simulink model "boostObserver_old"  (R2020a)
settings: Solver=VariableStepAuto  StartTime=0.0  StopTime=3.2  FixedStep=0.0005  MaxStep=9e-06  RelTol=1e-03  EnableMultiTasking=on
InitFcn:
  | kp=0.01;
  | ki=0.01;
  | 
  | k=2;
  | em=100000000;
  | GE=1/em;
  | GU=k*ki/GE;
  | GCE=k*kp/GU;
model workspace (MAT data in the model file):
  time = 0.8
values from neighbouring files (symbols this model uses):
  A1 = obj.boostConverter.A1    [BoostController.m]    (also in BoostConverter.m = [-obj.R/obj.L 0;0 -1/(obj.Ro*obj.C)]; BuckBoostConverter.m = [-obj.R/obj.L 0;0 -1/(obj.Ro*obj.C)]; obsmc.m = Asigma{1,1}; workspace_atual.mat = [-16.4  0; 0  -3.50877192982])
  A2 = obj.boostConverter.A2    [BoostController.m]    (also in BoostConverter.m = [-obj.R/obj.L -1/obj.L;1/obj.C -1/(obj.Ro*obj.C)]; BuckBoostConverter.m = [-obj.R/obj.L 1/obj.L;-1/obj.C -1/(obj.Ro*obj.C)]; obsmc.m = Asigma{1,2}; workspace_atual.mat = [-16.4  -200; 350.877192982  -3.50877192982])
  AlarmDeadTime = 0.50    (= 0.5)    [BoostFaultSimulation.m]    (also in workspace_atual.mat; workspace_certo.mat)
  B1 = obj.boostConverter.B1    [BoostController.m]    (also in BoostConverter.m = [1/obj.L;0]; BuckBoostConverter.m = [1/obj.L;0]; obsmc.m = Bsigma{1,1}; workspace_atual.mat = [200 0])
  boost_parameters = [obj.Ro,obj.R,obj.L,obj.C,obj.u]'    [BoostConverter.m]    (also in BuckBoostConverter.m; boostResults2Latex.m = boost.parameters(); workspace_atual.mat = [100 0.082 0.005 0.00285 190]; workspace_certo.mat = [100 0.082 0.005 0.00285 190])
  C = 1e-3    (= 0.001)    [boostResults2Latex.m]
  CiL = [0 1]    [workspace_atual.mat]    (also in workspace_certo.mat)
  Cmatrix = [1  0; 0  1]    [workspace_atual.mat]    (also in workspace_certo.mat)
  CVc = [1 0]    [workspace_atual.mat]    (also in workspace_certo.mat)
  D1 = [1  0; 0  1]    [workspace_atual.mat]    (also in workspace_certo.mat)
  FaultClass = 0    [BoostFaultSimulation.m]    (also in workspace_atual.mat = 1; workspace_certo.mat = 1)
  iLFaultSwitch = 0    [BoostFaultSimulation.m]    (also in workspace_atual.mat; workspace_certo.mat)
  iLFaultTime = 1.70    (= 1.7)    [BoostFaultSimulation.m]    (also in workspace_atual.mat; workspace_certo.mat)
  iLGainFaultFactor = 15    [BoostFaultSimulation.m]    (also in workspace_atual.mat; workspace_certo.mat)
  iLNoiseFaultSwitch = 0    [BoostFaultSimulation.m]    (also in workspace_atual.mat; workspace_certo.mat)
  iLNoiseTime = 1.70    (= 1.7)    [BoostFaultSimulation.m]    (also in workspace_atual.mat; workspace_certo.mat)
  Jth = 2000    [workspace_atual.mat]    (also in workspace_certo.mat)
  L = 1e-3    (= 0.001)    [boostResults2Latex.m]    (also in obsmc.m = sdpvar(3,1,'full'))
  LoadAddResistor = obj.LoadAddFactor*obj.Ro    [BoostFaultSimulation.m]    (also in workspace_atual.mat = 30; workspace_certo.mat = 30)
  LoadAddSignalSwitch = 1    [BoostFaultSimulation.m]    (also in workspace_atual.mat; workspace_certo.mat)
  LoadAddSwitch = 0    [BoostFaultSimulation.m]    (also in workspace_atual.mat; workspace_certo.mat)
  LoadAddTime = 0.90    (= 0.9)    [BoostFaultSimulation.m]    (also in workspace_atual.mat; workspace_certo.mat)
  LoadRemoveResistor = obj.Ro*(1-obj.LoadRemoveFactor)/(obj.LoadRemoveFactor)    [BoostFaultSimulation.m]    (also in workspace_atual.mat = 233.333333333; workspace_certo.mat = 233.333333333)
  LoadRemoveSignalSwitch = 1    [BoostFaultSimulation.m]    (also in workspace_atual.mat; workspace_certo.mat)
  LoadRemoveSwitch = 0    [BoostFaultSimulation.m]    (also in workspace_atual.mat; workspace_certo.mat)
  LoadRemoveTime = 0.90    (= 0.9)    [BoostFaultSimulation.m]    (also in workspace_atual.mat; workspace_certo.mat)
  LobsiL = [1737913.15707 66180.0912281]    [workspace_atual.mat]    (also in workspace_certo.mat)
  LobsVc = [61200 1]    [workspace_atual.mat]    (also in workspace_certo.mat)
  ObsEp = 70    [workspace_atual.mat]    (also in workspace_certo.mat)
  R = 0.1    [boostResults2Latex.m]    (also in workspace_atual.mat = 0.082; workspace_certo.mat = 0.082)
  ReconfigDelay = 0    [BoostFaultSimulation.m]    (also in workspace_atual.mat = 0.2; workspace_certo.mat = 0.2)
  ReconfigSwitch = 0    [BoostFaultSimulation.m]    (also in workspace_atual.mat; workspace_certo.mat)
  ReconfigTime = 1.707    [BoostFaultSimulation.m]    (also in workspace_atual.mat; workspace_certo.mat)
  rho = 5    [workspace_atual.mat]    (also in workspace_certo.mat)
  RMSfrequency = 47.61    [BoostFaultSimulation.m]    (also in workspace_atual.mat; workspace_certo.mat)
  Ro = 100    [BoostFaultSimulation.m]    (also in boostResults2Latex.m = 10; workspace_atual.mat; workspace_certo.mat)
  Smep = 80    [workspace_atual.mat]    (also in workspace_certo.mat)
  SourceAddSignalSwitch = 1    [BoostFaultSimulation.m]    (also in workspace_atual.mat; workspace_certo.mat)
  SourceAddSwitch = 0    [BoostFaultSimulation.m]    (also in workspace_atual.mat; workspace_certo.mat)
  SourceAddTime = 0.90    (= 0.9)    [BoostFaultSimulation.m]    (also in workspace_atual.mat; workspace_certo.mat)
  SourceAddVoltage = obj.SourceAddFactor*obj.u    [BoostFaultSimulation.m]    (also in workspace_atual.mat = 19; workspace_certo.mat = 19)
  SourceRemoveSignalSwitch = 1    [BoostFaultSimulation.m]    (also in workspace_atual.mat; workspace_certo.mat)
  SourceRemoveSwitch = 0    [BoostFaultSimulation.m]    (also in workspace_atual.mat; workspace_certo.mat)
  SourceRemoveTime = 0.90    (= 0.9)    [BoostFaultSimulation.m]    (also in workspace_atual.mat; workspace_certo.mat)
  SourceRemoveVoltage = obj.SourceRemoveFactor*obj.u    [BoostFaultSimulation.m]    (also in workspace_atual.mat = 19; workspace_certo.mat = 19)
  ueq = 0.5    [workspace_atual.mat]    (also in workspace_certo.mat)
  VcFaultSwitch = 0    [BoostFaultSimulation.m]    (also in workspace_atual.mat; workspace_certo.mat)
  VcFaultTime = 1.70    (= 1.7)    [BoostFaultSimulation.m]    (also in workspace_atual.mat; workspace_certo.mat)
  VcGainFaultFactor = 15    [BoostFaultSimulation.m]    (also in workspace_atual.mat; workspace_certo.mat)
  VcNoiseFaultSwitch = 0    [BoostFaultSimulation.m]    (also in workspace_atual.mat; workspace_certo.mat)
  VcNoiseTime = 1.70    (= 1.7)    [BoostFaultSimulation.m]    (also in workspace_atual.mat; workspace_certo.mat)
  ve = 380    [BoostFaultSimulation.m]    (also in boostResults2Latex.m = 100; workspace_atual.mat; workspace_certo.mat)
  x_e = [ie;ve]    [BoostConverter.m]    (also in BuckBoostConverter.m)
  xe = obj.boostConverter.equilibriumstate(ve)    [BoostController.m]    (also in workspace_atual.mat = [7.62509288104 380]; workspace_certo.mat = [7.62509288104 380])
undefined symbols (not defined in the file or in its folder): Atilde1, Atilde2, Ctilde1, Dtilde1, Dtilde2, F, G, MAXnet, MINnet
libraries: neural x74, powerlib x70, dspstat3 x16, simulink x9, powerlib_meascontrol x7, dspmtrx3 x7, dspmathops x3
(part 4 of 7)

== system boostObserver_old/reset/D(f_s)/Subsystem ==
  input : Inport
  FaultStep : Inport  Port=2
  NoiseStep : Inport  Port=3
  FaultSwtich : Inport  Port=4
  NoiseFaultSwitch : Inport  Port=5
  FaultFactor : Inport  Port=6
  Constant11 : Constant  Value=0
  Constant9 : Constant  Value=0
  Product : Product
  Subsystem : Subsystem
  Switch{9..11,13} (4 alike) : Switch  Criteria=u2 ~= 0
  iLFault Switch : MultiPortSwitch  DataPortOrder=Zero-based contiguous  DataPortForDefault=Additional data port  zeroidx=on
  output : Outport
  wires:
  input/1 -> Product/1, Switch11/3, Switch10/3, iLFault Switch/2, iLFault Switch/5
  Constant9/1 -> Switch10/1
  Switch13/1 -> Switch9/2
  Switch9/1 -> output/1
  Switch11/1 -> iLFault Switch/4
  Constant11/1 -> Switch13/3
  iLFault Switch/1 -> Switch9/3, Subsystem/1(input)
  Switch10/1 -> iLFault Switch/3
  FaultStep/1 -> Switch10/2, Switch11/2
  NoiseStep/1 -> Switch13/1
  FaultSwtich/1 -> iLFault Switch/1
  NoiseFaultSwitch/1 -> Switch13/2
  Product/1 -> Switch11/1
  FaultFactor/1 -> Product/2
  Subsystem/1(noiseOutput) -> Switch9/1

== system boostObserver_old/reset/D(f_s)/Subsystem2 ==
  input : Inport
  FaultStep : Inport  Port=2
  NoiseStep : Inport  Port=3
  FaultSwtich : Inport  Port=4
  NoiseFaultSwitch : Inport  Port=5
  FaultFactor : Inport  Port=6
  Constant11 : Constant  Value=0
  Constant9 : Constant  Value=0
  Product : Product
  Subsystem : Subsystem
  Switch10 : Switch  Criteria=u2 ~= 0
  Switch11 : Switch  Criteria=u2 ~= 0
  Switch13 : Switch  Criteria=u2 ~= 0
  Switch9 : Switch  Criteria=u2 ~= 0  ZeroCross=off
  iLFault Switch : MultiPortSwitch  DataPortOrder=Zero-based contiguous  DataPortForDefault=Additional data port  zeroidx=on
  output : Outport
  wires:
  input/1 -> Product/1, Switch11/3, iLFault Switch/2, Switch10/3, iLFault Switch/5
  Constant9/1 -> Switch10/1
  Switch13/1 -> Switch9/2
  Switch9/1 -> output/1
  Switch11/1 -> iLFault Switch/4
  Constant11/1 -> Switch13/3
  iLFault Switch/1 -> Switch9/3, Subsystem/1(input)
  Switch10/1 -> iLFault Switch/3
  FaultStep/1 -> Switch11/2, Switch10/2
  NoiseStep/1 -> Switch13/1
  FaultSwtich/1 -> iLFault Switch/1
  NoiseFaultSwitch/1 -> Switch13/2
  FaultFactor/1 -> Product/2
  Product/1 -> Switch11/1
  Subsystem/1(noiseOutput) -> Switch9/1

== system boostObserver_old/reset/ErrorGenerator/If Action Subsystem ==
  e_y : Inport
  Action Port : ActionPort  ActionPortLabel=if(u1 ~= 0)
  Matrix Multiply : Product  Multiplication=Matrix(*)
  Matrix Multiply1 : Product
  Matrizes A1 : Constant  Value=rho
  Matrizes A2 : Constant  Value=F
  Normalization : dspmathops/Normalization  NormType=2-norm  Bias=1e-10  NormOver=Each column  Dimension=1  roundingMode=Floor  overflowMode=off  accumDataTypeStr=Inherit: Same as product output  accumLastDataTypeStr=Inherit: Same as product output  outputDataTypeStr=Inherit: Same as product output  outputMin=[]  outputMax=[]  outputLastDataTypeStr=Inherit: Same as product output
  v : Outport
  wires:
  Matrix Multiply/1 -> Normalization/1
  Matrizes A2/1 -> Matrix Multiply/1
  Normalization/1 -> Matrix Multiply1/2
  e_y/1 -> Matrix Multiply/2
  Matrizes A1/1 -> Matrix Multiply1/1
  Matrix Multiply1/1 -> v/1

== system boostObserver_old/reset/ErrorGenerator/If Action Subsystem1 ==
  e_y : Inport
  Action Port : ActionPort  ActionPortLabel=else
  v : Outport
  wires:
  e_y/1 -> v/1

== system boostObserver_old/reset/Fault Identification Neural Netowrk/Pattern Recognition Neural Network2 ==
  Input : Inport  PortDimensions=3
      mask Display: e = 0.06;c1 = [120 230 180]/255;c2 = ([120 230 180]+0)/(256+128);c3 = ([120 230 180]+128)/(256+128);patch([0 1 1 0],[0 0 1 1],c1);patch([0 1 1 1-e 1-e 0+e],[0 0 1 1-e 0+e 0+e],c2);patch([0 0 1 1-e 0+e 0+e],[0 1 1 1-e 1-e 0+e],c3);plot([0 1 1 0 0],[0 0 1 1 0]);
  Layer 1 : Subsystem
      mask Display: e = 0.06;c1 = [120 150 230]/255;c2 = ([120 150 230]+0)/383;c3 = ([120 150 230]+128)/383;patch([0 1 1 0],[0 0 1 1],c1);patch([0 1 1 1-e 1-e 0+e],[0 0 1 1-e 0+e 0+e],c2);patch([0 0 1 1-e 0+e 0+e],[0 1 1 1-e 1-e 0+e],c3);plot([0 1 1 0 0],[0 0 1 1 0]);
  Layer 2 : Subsystem
      mask Display: e = 0.06;c1 = [120 150 230]/255;c2 = ([120 150 230]+0)/383;c3 = ([120 150 230]+128)/383;patch([0 1 1 0],[0 0 1 1],c1);patch([0 1 1 1-e 1-e 0+e],[0 0 1 1-e 0+e 0+e],c2);patch([0 0 1 1-e 0+e 0+e],[0 1 1 1-e 1-e 0+e],c3);plot([0 1 1 0 0],[0 0 1 1 0]);
  Process Input 1 : Subsystem
      mask Display: e = 0.06;c1 = [120 150 230]/255;c2 = ([120 150 230]+0)/383;c3 = ([120 150 230]+128)/383;patch([0 1 1 0],[0 0 1 1],c1);patch([0 1 1 1-e 1-e 0+e],[0 0 1 1-e 0+e 0+e],c2);patch([0 0 1 1-e 0+e 0+e],[0 1 1 1-e 1-e 0+e],c3);plot([0 1 1 0 0],[0 0 1 1 0]);
  Process Output 1 : Subsystem
      mask Display: e = 0.06;c1 = [120 150 230]/255;c2 = ([120 150 230]+0)/383;c3 = ([120 150 230]+128)/383;patch([0 1 1 0],[0 0 1 1],c1);patch([0 1 1 1-e 1-e 0+e],[0 0 1 1-e 0+e 0+e],c2);patch([0 0 1 1-e 0+e 0+e],[0 1 1 1-e 1-e 0+e],c3);plot([0 1 1 0 0],[0 0 1 1 0]);
  Output : Outport  InitialOutput=[0;0;0;0;0]
      mask Display: e = 0.06;c1 = [120 230 180]/255;c2 = ([120 230 180]+0)/(256+128);c3 = ([120 230 180]+128)/(256+128);patch([0 1 1 0],[0 0 1 1],c1);patch([0 1 1 1-e 1-e 0+e],[0 0 1 1-e 0+e 0+e],c2);patch([0 0 1 1-e 0+e 0+e],[0 1 1 1-e 1-e 0+e],c3);plot([0 1 1 0 0],[0 0 1 1 0]);
  wires:
  Input/1 -> Process Input 1/1(x)
  Process Output 1/1(y) -> Output/1
  Process Input 1/1(p) -> Layer 1/1("p{1}")
  Layer 1/1("a{1}") -> [feedback1]
  [feedback1] -> Layer 2/1("a{1} ")
  Layer 2/1("a{2}") -> Process Output 1/1(a)

== system boostObserver_old/reset/Fault Identification Neural Netowrk/Pattern Recognition Neural Network3 ==
  Input : Inport  PortDimensions=3
      mask Display: e = 0.06;c1 = [120 230 180]/255;c2 = ([120 230 180]+0)/(256+128);c3 = ([120 230 180]+128)/(256+128);patch([0 1 1 0],[0 0 1 1],c1);patch([0 1 1 1-e 1-e 0+e],[0 0 1 1-e 0+e 0+e],c2);patch([0 0 1 1-e 0+e 0+e],[0 1 1 1-e 1-e 0+e],c3);plot([0 1 1 0 0],[0 0 1 1 0]);
  Layer 1 : Subsystem
      mask Display: e = 0.06;c1 = [120 150 230]/255;c2 = ([120 150 230]+0)/383;c3 = ([120 150 230]+128)/383;patch([0 1 1 0],[0 0 1 1],c1);patch([0 1 1 1-e 1-e 0+e],[0 0 1 1-e 0+e 0+e],c2);patch([0 0 1 1-e 0+e 0+e],[0 1 1 1-e 1-e 0+e],c3);plot([0 1 1 0 0],[0 0 1 1 0]);
  Layer 2 : Subsystem
      mask Display: e = 0.06;c1 = [120 150 230]/255;c2 = ([120 150 230]+0)/383;c3 = ([120 150 230]+128)/383;patch([0 1 1 0],[0 0 1 1],c1);patch([0 1 1 1-e 1-e 0+e],[0 0 1 1-e 0+e 0+e],c2);patch([0 0 1 1-e 0+e 0+e],[0 1 1 1-e 1-e 0+e],c3);plot([0 1 1 0 0],[0 0 1 1 0]);
  Process Input 1 : Subsystem
      mask Display: e = 0.06;c1 = [120 150 230]/255;c2 = ([120 150 230]+0)/383;c3 = ([120 150 230]+128)/383;patch([0 1 1 0],[0 0 1 1],c1);patch([0 1 1 1-e 1-e 0+e],[0 0 1 1-e 0+e 0+e],c2);patch([0 0 1 1-e 0+e 0+e],[0 1 1 1-e 1-e 0+e],c3);plot([0 1 1 0 0],[0 0 1 1 0]);
  Process Output 1 : Subsystem
      mask Display: e = 0.06;c1 = [120 150 230]/255;c2 = ([120 150 230]+0)/383;c3 = ([120 150 230]+128)/383;patch([0 1 1 0],[0 0 1 1],c1);patch([0 1 1 1-e 1-e 0+e],[0 0 1 1-e 0+e 0+e],c2);patch([0 0 1 1-e 0+e 0+e],[0 1 1 1-e 1-e 0+e],c3);plot([0 1 1 0 0],[0 0 1 1 0]);
  Output : Outport  InitialOutput=[0;0;0;0;0]
      mask Display: e = 0.06;c1 = [120 230 180]/255;c2 = ([120 230 180]+0)/(256+128);c3 = ([120 230 180]+128)/(256+128);patch([0 1 1 0],[0 0 1 1],c1);patch([0 1 1 1-e 1-e 0+e],[0 0 1 1-e 0+e 0+e],c2);patch([0 0 1 1-e 0+e 0+e],[0 1 1 1-e 1-e 0+e],c3);plot([0 1 1 0 0],[0 0 1 1 0]);
  wires:
  Input/1 -> Process Input 1/1(x)
  Process Output 1/1(y) -> Output/1
  Process Input 1/1(p) -> Layer 1/1("p{1}")
  Layer 1/1("a{1}") -> [feedback1]
  [feedback1] -> Layer 2/1("a{1} ")
  Layer 2/1("a{2}") -> Process Output 1/1(a)

== system boostObserver_old/reset/If Action Subsystem1/GetInitialTime ==
  Clock : Inport
  Constant2 : Constant  Value=0
  Constant3 : Constant
  Constant4 : Constant  Value=0
  Edge Detector : powerlib_meascontrol/Logic/Edge Detector  model=Rising  ic=0  Ts=0
      settings: SourceProductBaseCode=PS
  If : If
  If Action Subsystem : Subsystem  TreatAsAtomicUnit=on
  If Action Subsystem1 : Subsystem  TreatAsAtomicUnit=on
  Memory : Memory
  Merge : Merge
  Switch : Switch  Criteria=u2 > Threshold
  Switch1 : Switch  Criteria=u2 > Threshold
  InitialTime : Outport
  wires:
  If/2 -> If Action Subsystem1/Action
  Memory/1 -> Switch1/3
  Constant3/1 -> Switch/1
  Switch1/1 -> InitialTime/1, Memory/1
  Merge/1 -> Switch1/2, Switch1/1
  Constant4/1 -> Switch/3
  Switch/1 -> If/1
  Constant2/1 -> If Action Subsystem1/1(In1)
  Clock/1 -> [Clock], Edge Detector/1
  If Action Subsystem/1(Out1) -> Merge/2
  Edge Detector/1 -> Switch/2
  [Clock] -> If Action Subsystem/1(In1)
  If/1 -> If Action Subsystem/Action
  If Action Subsystem1/1(Out1) -> Merge/1

== system boostObserver_old/reset/If Action Subsystem4/GetInitialTime ==
  Clock : Inport
  Constant2 : Constant  Value=0
  Constant3 : Constant
  Constant4 : Constant  Value=0
  Edge Detector : powerlib_meascontrol/Logic/Edge Detector  model=Rising  ic=0  Ts=0
      settings: SourceProductBaseCode=PS
  If : If
  If Action Subsystem : Subsystem  TreatAsAtomicUnit=on
  If Action Subsystem1 : Subsystem  TreatAsAtomicUnit=on
  Memory : Memory
  Merge : Merge
  Switch : Switch  Criteria=u2 > Threshold
  Switch1 : Switch  Criteria=u2 > Threshold
  InitialTime : Outport
  wires:
  If/2 -> If Action Subsystem1/Action
  Memory/1 -> Switch1/3
  Constant3/1 -> Switch/1
  Switch1/1 -> InitialTime/1, Memory/1
  Merge/1 -> Switch1/2, Switch1/1
  Constant4/1 -> Switch/3
  Switch/1 -> If/1
  Constant2/1 -> If Action Subsystem1/1(In1)
  Clock/1 -> [Clock], Edge Detector/1
  If Action Subsystem/1(Out1) -> Merge/2
  Edge Detector/1 -> Switch/2
  [Clock] -> If Action Subsystem/1(In1)
  If/1 -> If Action Subsystem/Action
  If Action Subsystem1/1(Out1) -> Merge/1

== system boostObserver_old/reset/Sliding Mode Observer 5/ObserverDynamics ==
  ey : Inport
  v : Inport  Port=2
  sigma : Inport  Port=3
  Gain : Gain  Gain=Atilde1  Multiplication=Matrix(K*u)
  Gain1 : Gain  Gain=G  Multiplication=Matrix(K*u)
  Gain3 : Gain  Gain=Dtilde1  Multiplication=Matrix(K*u)
  Gain5 : Gain  Gain=Atilde2  Multiplication=Matrix(K*u)
  Gain7 : Gain  Gain=Dtilde2  Multiplication=Matrix(K*u)
  Integral : Subsystem
  Sum : Sum  Inputs=|+++
  Sum1 : Sum  Inputs=|+++
  Switch1 : Switch  Criteria=u2 > Threshold
  e_tilde_hat : Outport
  wires:
  sigma/1 -> Switch1/2
  Switch1/1 -> Integral/1(e_hat_dot)  "v"
  Integral/1(e_hat) -> Gain/1, e_tilde_hat/1, Gain5/1
  ey/1 -> Gain1/1
  v/1 -> Gain7/1, Gain3/1
  Sum1/1 -> Switch1/3
  Sum/1 -> Switch1/1
  Gain7/1 -> Sum1/2
  Gain5/1 -> Sum1/3
  Gain3/1 -> Sum/1
  Gain1/1 -> Sum1/1, Sum/2
  Gain/1 -> Sum/3

== system boostObserver_old/reset/Subsystem/SlidingSurface ==
  S : Inport
  ep : Inport  Port=2
  Abs : Abs  ZeroCross=off
  GreaterThan : RelationalOperator  Operator=>  OutDataTypeStr=boolean  RndMeth=Simplest
  If : If  IfExpression=u1 ~= 0
  If Action Subsystem : Subsystem  TreatAsAtomicUnit=on
  If Action Subsystem2 : Subsystem  TreatAsAtomicUnit=on
  Merge1 : Merge
  d : Outport
  wires:
  If Action Subsystem2/1(d) -> Merge1/2
  [S] -> If Action Subsystem/1(S), If Action Subsystem2/1(S)
  If/2 -> If Action Subsystem2/Action
  If/1 -> If Action Subsystem/Action
  [ep] -> If Action Subsystem2/2(ep)
  S/1 -> [S], Abs/1
  If Action Subsystem/1(d) -> Merge1/1
  Abs/1 -> GreaterThan/1
  GreaterThan/1 -> If/1
  Merge1/1 -> d/1
  ep/1 -> [ep], GreaterThan/2

== system boostObserver_old/reset/Subsystem1/SlidingSurface ==
  S : Inport
  ep : Inport  Port=2
  Abs : Abs  ZeroCross=off
  GreaterThan : RelationalOperator  Operator=>  OutDataTypeStr=boolean  RndMeth=Simplest
  If : If  IfExpression=u1 ~= 0
  If Action Subsystem : Subsystem  TreatAsAtomicUnit=on
  If Action Subsystem2 : Subsystem  TreatAsAtomicUnit=on
  Merge1 : Merge
  d : Outport
  wires:
  If Action Subsystem2/1(d) -> Merge1/2
  [S] -> If Action Subsystem/1(S), If Action Subsystem2/1(S)
  If/2 -> If Action Subsystem2/Action
  If/1 -> If Action Subsystem/Action
  [ep] -> If Action Subsystem2/2(ep)
  S/1 -> [S], Abs/1
  If Action Subsystem/1(d) -> Merge1/1
  Abs/1 -> GreaterThan/1
  GreaterThan/1 -> If/1
  Merge1/1 -> d/1
  ep/1 -> [ep], GreaterThan/2

== system boostObserver_old/reset/Subsystem9/Residual Generator1 ==
  e_y : Inport
  Moving RMS : dspstat3/Moving RMS  Method=Sliding window  ForgettingFactorPort=off  SpecifyWindowLength=on  WindowLength=RMSfrequency  ForgettingFactor=0.9  SimulateUsing=Code generation
      settings: SourceProductBaseCode=DS
  RMS : Outport
  wires:
  e_y/1 -> Moving RMS/1
  Moving RMS/1 -> RMS/1

== system boostObserver_old/reset/Subsystem9/Residual Generator2 ==
  e_y : Inport
  Moving RMS : dspstat3/Moving RMS  Method=Sliding window  ForgettingFactorPort=off  SpecifyWindowLength=on  WindowLength=RMSfrequency  ForgettingFactor=0.9  SimulateUsing=Code generation
      settings: SourceProductBaseCode=DS
  RMS : Outport
  wires:
  e_y/1 -> Moving RMS/1
  Moving RMS/1 -> RMS/1

== system boostObserver_old/reset/Vc OBserver/calc_x_hat ==
  sigma : Inport
  rsign : Inport  Port=2
  Lobs : Inport  Port=3
  Gain : Gain  Gain=A1  Multiplication=Matrix(K*u)
  Gain5 : Gain  Gain=A2  Multiplication=Matrix(K*u)
  Integral : Subsystem
  Matrix Multiply : Product  Multiplication=Matrix(*)
  MatrizesA8 : Constant  Value=B1*u
  Scope1 : Scope
  Sum : Sum  Inputs=|+++
  Sum1 : Sum  Inputs=|+++
  Switch1 : Switch  Criteria=u2 ~= 0
  x_hat : Outport
  wires:
  sigma/1 -> Switch1/2
  Switch1/1 -> Integral/1(x_hat_dot)  "v"
  Integral/1(x_hat) -> Scope1/1, x_hat/1, Gain/1, Gain5/1
  Sum1/1 -> Switch1/3
  Sum/1 -> Switch1/1
  Gain/1 -> Sum/3
  Gain5/1 -> Sum1/3
  Matrix Multiply/1 -> Sum/2, Sum1/2
  MatrizesA8/1 -> Sum1/1, Sum/1
  Lobs/1 -> Matrix Multiply/1
  rsign/1 -> Matrix Multiply/2

== system boostObserver_old/reset/iL Observer/calc_x_hat ==
  sigma : Inport
  rsign : Inport  Port=2
  Lobs : Inport  Port=3
  Gain : Gain  Gain=A1  Multiplication=Matrix(K*u)
  Gain5 : Gain  Gain=A2  Multiplication=Matrix(K*u)
  Integral : Subsystem
  Matrix Multiply : Product  Multiplication=Matrix(*)
  MatrizesA8 : Constant  Value=B1*u
  Scope1 : Scope
  Sum : Sum  Inputs=|+++
  Sum1 : Sum  Inputs=|+++
  Switch1 : Switch  Criteria=u2 ~= 0
  x_hat : Outport
  wires:
  sigma/1 -> Switch1/2
  Switch1/1 -> Integral/1(x_hat_dot)  "v"
  Integral/1(x_hat) -> Scope1/1, x_hat/1, Gain/1, Gain5/1
  Sum1/1 -> Switch1/3
  Sum/1 -> Switch1/1
  Gain/1 -> Sum/3
  Gain5/1 -> Sum1/3
  Matrix Multiply/1 -> Sum/2, Sum1/2
  MatrizesA8/1 -> Sum1/1, Sum/1
  Lobs/1 -> Matrix Multiply/1
  rsign/1 -> Matrix Multiply/2

== system boostObserver_old/Subsystem/Boost Converter/TipoEntrada/disturbio ==
  Step1 : Step  SampleTime=0
  Step2 : Step  Time=1.1  After=-1  SampleTime=0
  Sum : Sum  Inputs=|++
  disturbio : Outport
  wires:
  Sum/1 -> disturbio/1
  Step2/1 -> Sum/2
  Step1/1 -> Sum/1

== system boostObserver_old/Subsystem/Boost Converter/TipoEntrada/disturbio1 ==
  Step1 : Step  Time=1.2  SampleTime=0
  Step2 : Step  Time=1.4  After=-1  SampleTime=0
  Sum : Sum  Inputs=|++
  disturbio : Outport
  wires:
  Sum/1 -> disturbio/1
  Step2/1 -> Sum/2
  Step1/1 -> Sum/1

== system boostObserver_old/Subsystem/Boost Converter/TipoEntrada/disturbio2 ==
  Step1 : Step  Time=1.2  SampleTime=0
  Step2 : Step  Time=1.4  After=-1  SampleTime=0
  Sum : Sum  Inputs=|++
  disturbio : Outport
  wires:
  Sum/1 -> disturbio/1
  Step2/1 -> Sum/2
  Step1/1 -> Sum/1

== system boostObserver_old/Subsystem/Boost Converter/TipoEntrada/disturbio3 ==
  Step1 : Step  SampleTime=0
  Step2 : Step  Time=1.1  After=-1  SampleTime=0
  Sum : Sum  Inputs=|++
  disturbio : Outport
  wires:
  Sum/1 -> disturbio/1
  Step2/1 -> Sum/2
  Step1/1 -> Sum/1

== system boostObserver_old/Subsystem/Controlador1/SlidingSurface/If Action Subsystem ==
  S : Inport
  Action Port : ActionPort  ActionPortLabel=if(u1 ~= 0)
  Sign : Signum
  d : Outport
  wires:
  S/1 -> Sign/1
  Sign/1 -> d/1

== system boostObserver_old/Subsystem/Controlador1/SlidingSurface/If Action Subsystem2 ==
  S : Inport
  ep : Inport  Port=2
  Action Port : ActionPort  ActionPortLabel=else
  Divide : Product  Inputs=*/
  d : Outport
  wires:
  S/1 -> Divide/1
  ep/1 -> Divide/2
  Divide/1 -> d/1

== system boostObserver_old/Subsystem/D(f_s)/Subsystem/Subsystem ==
  input : Inport
  Add : Sum
  Band-Limited White Noise : simulink/Sources/Band-Limited White Noise  Cov=[0.1]  Ts=0.1  seed=[23341]
  noiseOutput : Outport
  wires:
  Band-Limited White Noise/1 -> Add/1
  Add/1 -> noiseOutput/1
  input/1 -> Add/2

== system boostObserver_old/Subsystem/D(f_s)/Subsystem2/Subsystem ==
  input : Inport
  Add : Sum
  Band-Limited White Noise : simulink/Sources/Band-Limited White Noise  Cov=[0.1]  Ts=0.1  seed=[23341]
  noiseOutput : Outport
  wires:
  Band-Limited White Noise/1 -> Add/1
  Add/1 -> noiseOutput/1
  input/1 -> Add/2

== system boostObserver_old/Subsystem/Fault Identification Neural Netowrk/Pattern Recognition Neural Network1/Layer 1 ==
  "p{1}" : Inport  PortDimensions=3
      mask Display: e = 0.06;c1 = [120 230 180]/255;c2 = ([120 230 180]+0)/(256+128);c3 = ([120 230 180]+128)/(256+128);patch([0 1 1 0],[0 0 1 1],c1);patch([0 1 1 1-e 1-e 0+e],[0 0 1 1-e 0+e 0+e],c2);patch([0 0 1 1-e 0+e 0+e],[0 1 1 1-e 1-e 0+e],c3);plot([0 1 1 0 0],[0 0 1 1 0]);
  Delays 1 : Subsystem
      mask Display: e = 0.06;c1 = [120 150 230]/255;c2 = ([120 150 230]+0)/383;c3 = ([120 150 230]+128)/383;patch([0 1 1 0],[0 0 1 1],c1);patch([0 1 1 1-e 1-e 0+e],[0 0 1 1-e 0+e 0+e],c2);patch([0 0 1 1-e 0+e 0+e],[0 1 1 1-e 1-e 0+e],c3);plot([0 1 1 0 0],[0 0 1 1 0]);disp('0');
  "IW{1,1}" : Subsystem
      mask Display: e = 0.06;c1 = [120 150 230]/255;c2 = ([120 150 230]+0)/383;c3 = ([120 150 230]+128)/383;patch([0 1 1 0],[0 0 1 1],c1);patch([0 1 1 1-e 1-e 0+e],[0 0 1 1-e 0+e 0+e],c2);patch([0 0 1 1-e 0+e 0+e],[0 1 1 1-e 1-e 0+e],c3);plot([0 1 1 0 0],[0 0 1 1 0]);disp('W');
  "b{1}" : Constant  Value=[-3.0907169643136906955760423443280160427093505859375;-8.5532408660313894444016113993711769580841064453125;26.179031484954197850356649723835289478302001953125;0.130591451617109999272514642143505625426769256591796875]
      mask Display: e = 0.06;c1 = [120 150 230]/255;c2 = ([120 150 230]+0)/383;c3 = ([120 150 230]+128)/383;patch([0 1 1 0],[0 0 1 1],c1);patch([0 1 1 1-e 1-e 0+e],[0 0 1 1-e 0+e 0+e],c2);patch([0 0 1 1-e 0+e 0+e],[0 1 1 1-e 1-e 0+e],c3);plot([0 1 1 0 0],[0 0 1 1 0]);disp('b');
  netsum : Sum  Inputs=2  InputSameDT=on  SaturateOnIntegerOverflow=on  OutDataTypeStr=Inherit: Same as first input
      mask Display: e = 0.06;c1 = [120 150 230]/255;c2 = ([120 150 230]+0)/383;c3 = ([120 150 230]+128)/383;patch([0 1 1 0],[0 0 1 1],c1);patch([0 1 1 1-e 1-e 0+e],[0 0 1 1-e 0+e 0+e],c2);patch([0 0 1 1-e 0+e 0+e],[0 1 1 1-e 1-e 0+e],c3);plot([0 1 1 0 0],[0 0 1 1 0]);disp('+');
  tansig : neural/Transfer Functions/tansig
  "a{1}" : Outport  InitialOutput=[0;0;0;0]
      mask Display: e = 0.06;c1 = [120 230 180]/255;c2 = ([120 230 180]+0)/(256+128);c3 = ([120 230 180]+128)/(256+128);patch([0 1 1 0],[0 0 1 1],c1);patch([0 1 1 1-e 1-e 0+e],[0 0 1 1-e 0+e 0+e],c2);patch([0 0 1 1-e 0+e 0+e],[0 1 1 1-e 1-e 0+e],c3);plot([0 1 1 0 0],[0 0 1 1 0]);
  wires:
  "p{1}"/1 -> Delays 1/1("p{1}")
  Delays 1/1("pd{1,1}") -> "IW{1,1}"/1("pd{1,1}")
  "IW{1,1}"/1("iz{1,1}") -> netsum/1
  "b{1}"/1 -> netsum/2
  netsum/1 -> tansig/1
  tansig/1 -> "a{1}"/1

== system boostObserver_old/Subsystem/Fault Identification Neural Netowrk/Pattern Recognition Neural Network1/Layer 2 ==
  "a{1} " : Inport  PortDimensions=4
      mask Display: e = 0.06;c1 = [120 230 180]/255;c2 = ([120 230 180]+0)/(256+128);c3 = ([120 230 180]+128)/(256+128);patch([0 1 1 0],[0 0 1 1],c1);patch([0 1 1 1-e 1-e 0+e],[0 0 1 1-e 0+e 0+e],c2);patch([0 0 1 1-e 0+e 0+e],[0 1 1 1-e 1-e 0+e],c3);plot([0 1 1 0 0],[0 0 1 1 0]);
  Delays 1 : Subsystem
      mask Display: e = 0.06;c1 = [120 150 230]/255;c2 = ([120 150 230]+0)/383;c3 = ([120 150 230]+128)/383;patch([0 1 1 0],[0 0 1 1],c1);patch([0 1 1 1-e 1-e 0+e],[0 0 1 1-e 0+e 0+e],c2);patch([0 0 1 1-e 0+e 0+e],[0 1 1 1-e 1-e 0+e],c3);plot([0 1 1 0 0],[0 0 1 1 0]);disp('0');
  "LW{2,1}" : Subsystem
      mask Display: e = 0.06;c1 = [120 150 230]/255;c2 = ([120 150 230]+0)/383;c3 = ([120 150 230]+128)/383;patch([0 1 1 0],[0 0 1 1],c1);patch([0 1 1 1-e 1-e 0+e],[0 0 1 1-e 0+e 0+e],c2);patch([0 0 1 1-e 0+e 0+e],[0 1 1 1-e 1-e 0+e],c3);plot([0 1 1 0 0],[0 0 1 1 0]);disp('W');
  "b{2}" : Constant  Value=[-2.302427575546979188203522426192648708820343017578125;-5.91134493996858534359262193902395665645599365234375;6.8980698616354221286428582970984280109405517578125;0.77959090259712271464564992129453457891941070556640625;-0.782333279931369585113998255110345780849456787109375]
      mask Display: e = 0.06;c1 = [120 150 230]/255;c2 = ([120 150 230]+0)/383;c3 = ([120 150 230]+128)/383;patch([0 1 1 0],[0 0 1 1],c1);patch([0 1 1 1-e 1-e 0+e],[0 0 1 1-e 0+e 0+e],c2);patch([0 0 1 1-e 0+e 0+e],[0 1 1 1-e 1-e 0+e],c3);plot([0 1 1 0 0],[0 0 1 1 0]);disp('b');
  netsum : Sum  Inputs=2  InputSameDT=on  SaturateOnIntegerOverflow=on  OutDataTypeStr=Inherit: Same as first input
      mask Display: e = 0.06;c1 = [120 150 230]/255;c2 = ([120 150 230]+0)/383;c3 = ([120 150 230]+128)/383;patch([0 1 1 0],[0 0 1 1],c1);patch([0 1 1 1-e 1-e 0+e],[0 0 1 1-e 0+e 0+e],c2);patch([0 0 1 1-e 0+e 0+e],[0 1 1 1-e 1-e 0+e],c3);plot([0 1 1 0 0],[0 0 1 1 0]);disp('+');
  softmax : neural/Transfer Functions/softmax
      settings: SourceProductBaseCode=NN
  "a{2}" : Outport  InitialOutput=[0;0;0;0;0]
      mask Display: e = 0.06;c1 = [120 230 180]/255;c2 = ([120 230 180]+0)/(256+128);c3 = ([120 230 180]+128)/(256+128);patch([0 1 1 0],[0 0 1 1],c1);patch([0 1 1 1-e 1-e 0+e],[0 0 1 1-e 0+e 0+e],c2);patch([0 0 1 1-e 0+e 0+e],[0 1 1 1-e 1-e 0+e],c3);plot([0 1 1 0 0],[0 0 1 1 0]);
  wires:
  "a{1} "/1 -> Delays 1/1("p{2}")
  Delays 1/1("pd{2,1}") -> "LW{2,1}"/1("ad{2,1}")
  "LW{2,1}"/1("lz{2,1}") -> netsum/1
  "b{2}"/1 -> netsum/2
  netsum/1 -> softmax/1
  softmax/1 -> "a{2}"/1

== system boostObserver_old/Subsystem/Fault Identification Neural Netowrk/Pattern Recognition Neural Network1/Process Input 1 ==
  x : Inport  PortDimensions=3
      mask Display: e = 0.06;c1 = [120 230 180]/255;c2 = ([120 230 180]+0)/(256+128);c3 = ([120 230 180]+128)/(256+128);patch([0 1 1 0],[0 0 1 1],c1);patch([0 1 1 1-e 1-e 0+e],[0 0 1 1-e 0+e 0+e],c2);patch([0 0 1 1-e 0+e 0+e],[0 1 1 1-e 1-e 0+e],c3);plot([0 1 1 0 0],[0 0 1 1 0]);
  mapminmax : neural/Processing Functions/mapminmax  xmin=[0;0;-2641.94920061935135890962556005]  xmax=[786.388396902503131968842353672;8926.40391005816127290017902851;8647.99703455211783875711262226]  ymin=-1  ymax=1
  p : Outport  PortDimensions=3
      mask Display: e = 0.06;c1 = [120 230 180]/255;c2 = ([120 230 180]+0)/(256+128);c3 = ([120 230 180]+128)/(256+128);patch([0 1 1 0],[0 0 1 1],c1);patch([0 1 1 1-e 1-e 0+e],[0 0 1 1-e 0+e 0+e],c2);patch([0 0 1 1-e 0+e 0+e],[0 1 1 1-e 1-e 0+e],c3);plot([0 1 1 0 0],[0 0 1 1 0]);
  wires:
  x/1 -> mapminmax/1
  mapminmax/1 -> p/1

== system boostObserver_old/Subsystem/Fault Identification Neural Netowrk/Pattern Recognition Neural Network1/Process Output 1 ==
  a : Inport  PortDimensions=5
      mask Display: e = 0.06;c1 = [120 230 180]/255;c2 = ([120 230 180]+0)/(256+128);c3 = ([120 230 180]+128)/(256+128);patch([0 1 1 0],[0 0 1 1],c1);patch([0 1 1 1-e 1-e 0+e],[0 0 1 1-e 0+e 0+e],c2);patch([0 0 1 1-e 0+e 0+e],[0 1 1 1-e 1-e 0+e],c3);plot([0 1 1 0 0],[0 0 1 1 0]);
  y : Outport  PortDimensions=5
      mask Display: e = 0.06;c1 = [120 230 180]/255;c2 = ([120 230 180]+0)/(256+128);c3 = ([120 230 180]+128)/(256+128);patch([0 1 1 0],[0 0 1 1],c1);patch([0 1 1 1-e 1-e 0+e],[0 0 1 1-e 0+e 0+e],c2);patch([0 0 1 1-e 0+e 0+e],[0 1 1 1-e 1-e 0+e],c3);plot([0 1 1 0 0],[0 0 1 1 0]);
  wires:
  a/1 -> y/1

== system boostObserver_old/Subsystem/Sliding Mode Observer 5/ObserverDynamics/Integral ==
  e_hat_dot : Inport
  Ground{1..4} (4 alike) : Ground
  IC : InitialCondition  Value=[-xe;0;0]
  Integrator5 : Integrator  InitialConditionSource=external  InitialCondition=[-x_e; 0; 0]
  Mux : Mux
  e_hat : Outport
  wires:
  e_hat_dot/1 -> Integrator5/1
  Integrator5/1 -> e_hat/1
  IC/1 -> Integrator5/2
  Ground1/1 -> Mux/1
  Ground2/1 -> Mux/2
  Ground3/1 -> Mux/3
  Ground4/1 -> Mux/4
  Mux/1 -> IC/1

== system boostObserver_old/Subsystem/Subsystem/SlidingSurface/If Action Subsystem ==
  S : Inport
  Action Port : ActionPort  ActionPortLabel=if(u1 ~= 0)
  Sign : Signum
  d : Outport
  wires:
  S/1 -> Sign/1
  Sign/1 -> d/1

== system boostObserver_old/Subsystem/Subsystem/SlidingSurface/If Action Subsystem2 ==
  S : Inport
  ep : Inport  Port=2
  Action Port : ActionPort  ActionPortLabel=else
  Divide : Product  Inputs=*/
  d : Outport
  wires:
  S/1 -> Divide/1
  ep/1 -> Divide/2
  Divide/1 -> d/1

== system boostObserver_old/Subsystem/Subsystem1/SlidingSurface/If Action Subsystem ==
  S : Inport
  Action Port : ActionPort  ActionPortLabel=if(u1 ~= 0)
  Sign : Signum
  d : Outport
  wires:
  S/1 -> Sign/1
  Sign/1 -> d/1

== system boostObserver_old/Subsystem/Subsystem1/SlidingSurface/If Action Subsystem2 ==
  S : Inport
  ep : Inport  Port=2
  Action Port : ActionPort  ActionPortLabel=else
  Divide : Product  Inputs=*/
  d : Outport
  wires:
  S/1 -> Divide/1
  ep/1 -> Divide/2
  Divide/1 -> d/1

== system boostObserver_old/Subsystem/Vc OBserver/calc_x_hat/Integral ==
  x_hat_dot : Inport
  Ground1 : Ground
  Ground2 : Ground
  IC : InitialCondition  Value=[0;0]
  Integrator1 : Integrator  InitialConditionSource=external  InitialCondition=[-x_e; 0; 0]
  Mux : Mux  Inputs=2
  x_hat : Outport
  wires:
  x_hat_dot/1 -> Integrator1/1
  Integrator1/1 -> x_hat/1
  IC/1 -> Integrator1/2
  Ground1/1 -> Mux/1
  Ground2/1 -> Mux/2
  Mux/1 -> IC/1

== system boostObserver_old/Subsystem/iL Observer/calc_x_hat/Integral ==
  x_hat_dot : Inport
  Ground : Ground
  Ground1 : Ground
  IC : InitialCondition  Value=[0;0]
  Integrator1 : Integrator  InitialConditionSource=external  InitialCondition=[-x_e; 0; 0]
  Mux : Mux  Inputs=2
  x_hat : Outport
  wires:
  x_hat_dot/1 -> Integrator1/1
  Integrator1/1 -> x_hat/1
  Mux/1 -> IC/1
  Ground/1 -> Mux/1
  Ground1/1 -> Mux/2
  IC/1 -> Integrator1/2

== system boostObserver_old/Subsystem3/Boost Converter/TipoEntrada/disturbio ==
  Step1 : Step  SampleTime=0
  Step2 : Step  Time=1.1  After=-1  SampleTime=0
  Sum : Sum  Inputs=|++
  disturbio : Outport
  wires:
  Sum/1 -> disturbio/1
  Step2/1 -> Sum/2
  Step1/1 -> Sum/1

== system boostObserver_old/Subsystem3/Boost Converter/TipoEntrada/disturbio1 ==
  Step1 : Step  Time=1.2  SampleTime=0
  Step2 : Step  Time=1.4  After=-1  SampleTime=0
  Sum : Sum  Inputs=|++
  disturbio : Outport
  wires:
  Sum/1 -> disturbio/1
  Step2/1 -> Sum/2
  Step1/1 -> Sum/1

== system boostObserver_old/Subsystem3/Boost Converter/TipoEntrada/disturbio2 ==
  Step1 : Step  Time=1.2  SampleTime=0
  Step2 : Step  Time=1.4  After=-1  SampleTime=0
  Sum : Sum  Inputs=|++
  disturbio : Outport
  wires:
  Sum/1 -> disturbio/1
  Step2/1 -> Sum/2
  Step1/1 -> Sum/1

== system boostObserver_old/Subsystem3/Boost Converter/TipoEntrada/disturbio3 ==
  Step1 : Step  SampleTime=0
  Step2 : Step  Time=1.1  After=-1  SampleTime=0
  Sum : Sum  Inputs=|++
  disturbio : Outport
  wires:
  Sum/1 -> disturbio/1
  Step2/1 -> Sum/2
  Step1/1 -> Sum/1

== system boostObserver_old/Subsystem3/Controlador1/SlidingSurface/If Action Subsystem ==
  S : Inport
  Action Port : ActionPort
  Sign : Signum
  d : Outport
  wires:
  S/1 -> Sign/1
  Sign/1 -> d/1

== system boostObserver_old/Subsystem3/Controlador1/SlidingSurface/If Action Subsystem2 ==
  S : Inport
  ep : Inport  Port=2
  Action Port : ActionPort
  Divide : Product  Inputs=*/
  d : Outport
  wires:
  S/1 -> Divide/1
  ep/1 -> Divide/2
  Divide/1 -> d/1

== system boostObserver_old/Subsystem3/D(f_s)/Subsystem/Subsystem ==
  input : Inport
  Add : Sum
  Band-Limited White Noise : simulink/Sources/Band-Limited White Noise  Cov=[0.1]  Ts=0.1  seed=[23341]
  noiseOutput : Outport
  wires:
  Band-Limited White Noise/1 -> Add/1
  Add/1 -> noiseOutput/1
  input/1 -> Add/2

== system boostObserver_old/Subsystem3/D(f_s)/Subsystem2/Subsystem ==
  input : Inport
  Add : Sum
  Band-Limited White Noise : simulink/Sources/Band-Limited White Noise  Cov=[0.1]  Ts=0.1  seed=[23341]
  noiseOutput : Outport
  wires:
  Band-Limited White Noise/1 -> Add/1
  Add/1 -> noiseOutput/1
  input/1 -> Add/2

== system boostObserver_old/Subsystem3/Fault Identification Neural Netowrk/Pattern Recognition Neural Network/Layer 1 ==
  "p{1}" : Inport  PortDimensions=3
      mask Display: e = 0.06;c1 = [120 230 180]/255;c2 = ([120 230 180]+0)/(256+128);c3 = ([120 230 180]+128)/(256+128);patch([0 1 1 0],[0 0 1 1],c1);patch([0 1 1 1-e 1-e 0+e],[0 0 1 1-e 0+e 0+e],c2);patch([0 0 1 1-e 0+e 0+e],[0 1 1 1-e 1-e 0+e],c3);plot([0 1 1 0 0],[0 0 1 1 0]);
  Delays 1 : Subsystem
      mask Display: e = 0.06;c1 = [120 150 230]/255;c2 = ([120 150 230]+0)/383;c3 = ([120 150 230]+128)/383;patch([0 1 1 0],[0 0 1 1],c1);patch([0 1 1 1-e 1-e 0+e],[0 0 1 1-e 0+e 0+e],c2);patch([0 0 1 1-e 0+e 0+e],[0 1 1 1-e 1-e 0+e],c3);plot([0 1 1 0 0],[0 0 1 1 0]);disp('0');
  "IW{1,1}" : Subsystem
      mask Display: e = 0.06;c1 = [120 150 230]/255;c2 = ([120 150 230]+0)/383;c3 = ([120 150 230]+128)/383;patch([0 1 1 0],[0 0 1 1],c1);patch([0 1 1 1-e 1-e 0+e],[0 0 1 1-e 0+e 0+e],c2);patch([0 0 1 1-e 0+e 0+e],[0 1 1 1-e 1-e 0+e],c3);plot([0 1 1 0 0],[0 0 1 1 0]);disp('W');
  "b{1}" : Constant  Value=[-2.847316574931408439397273468784987926483154296875;1.842175672727865087807685995358042418956756591796875;2.933131194349774428786759017384611070156097412109375;-10.693084308006490346087957732379436492919921875;-8.571133472089218940936916624195873737335205078125;1.667012626659359231240387089201249182224273681640625;2.875884206192194536555462036631070077419281005859375]
      mask Display: e = 0.06;c1 = [120 150 230]/255;c2 = ([120 150 230]+0)/383;c3 = ([120 150 230]+128)/383;patch([0 1 1 0],[0 0 1 1],c1);patch([0 1 1 1-e 1-e 0+e],[0 0 1 1-e 0+e 0+e],c2);patch([0 0 1 1-e 0+e 0+e],[0 1 1 1-e 1-e 0+e],c3);plot([0 1 1 0 0],[0 0 1 1 0]);disp('b');
  netsum : Sum  Inputs=2  InputSameDT=on  SaturateOnIntegerOverflow=on  OutDataTypeStr=Inherit: Same as first input
      mask Display: e = 0.06;c1 = [120 150 230]/255;c2 = ([120 150 230]+0)/383;c3 = ([120 150 230]+128)/383;patch([0 1 1 0],[0 0 1 1],c1);patch([0 1 1 1-e 1-e 0+e],[0 0 1 1-e 0+e 0+e],c2);patch([0 0 1 1-e 0+e 0+e],[0 1 1 1-e 1-e 0+e],c3);plot([0 1 1 0 0],[0 0 1 1 0]);disp('+');
  tansig : neural/Transfer Functions/tansig
  "a{1}" : Outport  InitialOutput=[0;0;0;0;0;0;0]
      mask Display: e = 0.06;c1 = [120 230 180]/255;c2 = ([120 230 180]+0)/(256+128);c3 = ([120 230 180]+128)/(256+128);patch([0 1 1 0],[0 0 1 1],c1);patch([0 1 1 1-e 1-e 0+e],[0 0 1 1-e 0+e 0+e],c2);patch([0 0 1 1-e 0+e 0+e],[0 1 1 1-e 1-e 0+e],c3);plot([0 1 1 0 0],[0 0 1 1 0]);
  wires:
  "p{1}"/1 -> Delays 1/1("p{1}")
  Delays 1/1("pd{1,1}") -> "IW{1,1}"/1("pd{1,1}")
  "IW{1,1}"/1("iz{1,1}") -> netsum/1
  "b{1}"/1 -> netsum/2
  netsum/1 -> tansig/1
  tansig/1 -> "a{1}"/1

== system boostObserver_old/Subsystem3/Fault Identification Neural Netowrk/Pattern Recognition Neural Network/Layer 2 ==
  "a{1} " : Inport  PortDimensions=7
      mask Display: e = 0.06;c1 = [120 230 180]/255;c2 = ([120 230 180]+0)/(256+128);c3 = ([120 230 180]+128)/(256+128);patch([0 1 1 0],[0 0 1 1],c1);patch([0 1 1 1-e 1-e 0+e],[0 0 1 1-e 0+e 0+e],c2);patch([0 0 1 1-e 0+e 0+e],[0 1 1 1-e 1-e 0+e],c3);plot([0 1 1 0 0],[0 0 1 1 0]);
  Delays 1 : Subsystem
      mask Display: e = 0.06;c1 = [120 150 230]/255;c2 = ([120 150 230]+0)/383;c3 = ([120 150 230]+128)/383;patch([0 1 1 0],[0 0 1 1],c1);patch([0 1 1 1-e 1-e 0+e],[0 0 1 1-e 0+e 0+e],c2);patch([0 0 1 1-e 0+e 0+e],[0 1 1 1-e 1-e 0+e],c3);plot([0 1 1 0 0],[0 0 1 1 0]);disp('0');
  "LW{2,1}" : Subsystem
      mask Display: e = 0.06;c1 = [120 150 230]/255;c2 = ([120 150 230]+0)/383;c3 = ([120 150 230]+128)/383;patch([0 1 1 0],[0 0 1 1],c1);patch([0 1 1 1-e 1-e 0+e],[0 0 1 1-e 0+e 0+e],c2);patch([0 0 1 1-e 0+e 0+e],[0 1 1 1-e 1-e 0+e],c3);plot([0 1 1 0 0],[0 0 1 1 0]);disp('W');
  "b{2}" : Constant  Value=[1.5644619115450904001107801377656869590282440185546875;-1.983017578427060723100794348283670842647552490234375;0.385171036103830688457350106546073220670223236083984375;-0.041263748126133668880921590016441768966615200042724609375;-1.52556283987809226942999885068275034427642822265625;0.91786543306534340569413643606822006404399871826171875]
      mask Display: e = 0.06;c1 = [120 150 230]/255;c2 = ([120 150 230]+0)/383;c3 = ([120 150 230]+128)/383;patch([0 1 1 0],[0 0 1 1],c1);patch([0 1 1 1-e 1-e 0+e],[0 0 1 1-e 0+e 0+e],c2);patch([0 0 1 1-e 0+e 0+e],[0 1 1 1-e 1-e 0+e],c3);plot([0 1 1 0 0],[0 0 1 1 0]);disp('b');
  netsum : Sum  Inputs=2  InputSameDT=on  SaturateOnIntegerOverflow=on  OutDataTypeStr=Inherit: Same as first input
      mask Display: e = 0.06;c1 = [120 150 230]/255;c2 = ([120 150 230]+0)/383;c3 = ([120 150 230]+128)/383;patch([0 1 1 0],[0 0 1 1],c1);patch([0 1 1 1-e 1-e 0+e],[0 0 1 1-e 0+e 0+e],c2);patch([0 0 1 1-e 0+e 0+e],[0 1 1 1-e 1-e 0+e],c3);plot([0 1 1 0 0],[0 0 1 1 0]);disp('+');
  softmax : neural/Transfer Functions/softmax
      settings: SourceProductBaseCode=NN
  "a{2}" : Outport  InitialOutput=[0;0;0;0;0;0]
      mask Display: e = 0.06;c1 = [120 230 180]/255;c2 = ([120 230 180]+0)/(256+128);c3 = ([120 230 180]+128)/(256+128);patch([0 1 1 0],[0 0 1 1],c1);patch([0 1 1 1-e 1-e 0+e],[0 0 1 1-e 0+e 0+e],c2);patch([0 0 1 1-e 0+e 0+e],[0 1 1 1-e 1-e 0+e],c3);plot([0 1 1 0 0],[0 0 1 1 0]);
  wires:
  "a{1} "/1 -> Delays 1/1("p{2}")
  Delays 1/1("pd{2,1}") -> "LW{2,1}"/1("ad{2,1}")
  "LW{2,1}"/1("lz{2,1}") -> netsum/1
  "b{2}"/1 -> netsum/2
  netsum/1 -> softmax/1
  softmax/1 -> "a{2}"/1

== system boostObserver_old/Subsystem3/Fault Identification Neural Netowrk/Pattern Recognition Neural Network/Process Input 1 ==
  x : Inport  PortDimensions=3
      mask Display: e = 0.06;c1 = [120 230 180]/255;c2 = ([120 230 180]+0)/(256+128);c3 = ([120 230 180]+128)/(256+128);patch([0 1 1 0],[0 0 1 1],c1);patch([0 1 1 1-e 1-e 0+e],[0 0 1 1-e 0+e 0+e],c2);patch([0 0 1 1-e 0+e 0+e],[0 1 1 1-e 1-e 0+e],c3);plot([0 1 1 0 0],[0 0 1 1 0]);
  mapminmax : neural/Processing Functions/mapminmax  xmin=[0;0;0]  xmax=[555.172023885883049842959735543;9710.23056441231165081262588501;572.471571737876956831314601004]  ymin=-1  ymax=1
  p : Outport  PortDimensions=3
      mask Display: e = 0.06;c1 = [120 230 180]/255;c2 = ([120 230 180]+0)/(256+128);c3 = ([120 230 180]+128)/(256+128);patch([0 1 1 0],[0 0 1 1],c1);patch([0 1 1 1-e 1-e 0+e],[0 0 1 1-e 0+e 0+e],c2);patch([0 0 1 1-e 0+e 0+e],[0 1 1 1-e 1-e 0+e],c3);plot([0 1 1 0 0],[0 0 1 1 0]);
  wires:
  x/1 -> mapminmax/1
  mapminmax/1 -> p/1

== system boostObserver_old/Subsystem3/Fault Identification Neural Netowrk/Pattern Recognition Neural Network/Process Output 1 ==
  a : Inport  PortDimensions=6
      mask Display: e = 0.06;c1 = [120 230 180]/255;c2 = ([120 230 180]+0)/(256+128);c3 = ([120 230 180]+128)/(256+128);patch([0 1 1 0],[0 0 1 1],c1);patch([0 1 1 1-e 1-e 0+e],[0 0 1 1-e 0+e 0+e],c2);patch([0 0 1 1-e 0+e 0+e],[0 1 1 1-e 1-e 0+e],c3);plot([0 1 1 0 0],[0 0 1 1 0]);
  y : Outport  PortDimensions=6
      mask Display: e = 0.06;c1 = [120 230 180]/255;c2 = ([120 230 180]+0)/(256+128);c3 = ([120 230 180]+128)/(256+128);patch([0 1 1 0],[0 0 1 1],c1);patch([0 1 1 1-e 1-e 0+e],[0 0 1 1-e 0+e 0+e],c2);patch([0 0 1 1-e 0+e 0+e],[0 1 1 1-e 1-e 0+e],c3);plot([0 1 1 0 0],[0 0 1 1 0]);
  wires:
  a/1 -> y/1

== system boostObserver_old/Subsystem3/Fault Identification Neural Netowrk/Pattern Recognition Neural Network Reconfig Big Data/Layer 1 ==
  "p{1}" : Inport  PortDimensions=3
      mask Display: e = 0.06;c1 = [120 230 180]/255;c2 = ([120 230 180]+0)/(256+128);c3 = ([120 230 180]+128)/(256+128);patch([0 1 1 0],[0 0 1 1],c1);patch([0 1 1 1-e 1-e 0+e],[0 0 1 1-e 0+e 0+e],c2);patch([0 0 1 1-e 0+e 0+e],[0 1 1 1-e 1-e 0+e],c3);plot([0 1 1 0 0],[0 0 1 1 0]);
  Delays 1 : Subsystem
      mask Display: e = 0.06;c1 = [120 150 230]/255;c2 = ([120 150 230]+0)/383;c3 = ([120 150 230]+128)/383;patch([0 1 1 0],[0 0 1 1],c1);patch([0 1 1 1-e 1-e 0+e],[0 0 1 1-e 0+e 0+e],c2);patch([0 0 1 1-e 0+e 0+e],[0 1 1 1-e 1-e 0+e],c3);plot([0 1 1 0 0],[0 0 1 1 0]);disp('0');
  "IW{1,1}" : Subsystem
      mask Display: e = 0.06;c1 = [120 150 230]/255;c2 = ([120 150 230]+0)/383;c3 = ([120 150 230]+128)/383;patch([0 1 1 0],[0 0 1 1],c1);patch([0 1 1 1-e 1-e 0+e],[0 0 1 1-e 0+e 0+e],c2);patch([0 0 1 1-e 0+e 0+e],[0 1 1 1-e 1-e 0+e],c3);plot([0 1 1 0 0],[0 0 1 1 0]);disp('W');
  "b{1}" : Constant  Value=[-2.68966835194885955928612020215950906276702880859375;2.647773460815799229095546252210624516010284423828125;5.124333684580253844842445687390863895416259765625;0.72318417747872654199881026215734891593456268310546875;0.84991434193365922311613758211024105548858642578125;-6.36145574283156722827925477758981287479400634765625;-9.7283675351101965844691221718676388263702392578125]
      mask Display: e = 0.06;c1 = [120 150 230]/255;c2 = ([120 150 230]+0)/383;c3 = ([120 150 230]+128)/383;patch([0 1 1 0],[0 0 1 1],c1);patch([0 1 1 1-e 1-e 0+e],[0 0 1 1-e 0+e 0+e],c2);patch([0 0 1 1-e 0+e 0+e],[0 1 1 1-e 1-e 0+e],c3);plot([0 1 1 0 0],[0 0 1 1 0]);disp('b');
  netsum : Sum  Inputs=2  InputSameDT=on  SaturateOnIntegerOverflow=on  OutDataTypeStr=Inherit: Same as first input
      mask Display: e = 0.06;c1 = [120 150 230]/255;c2 = ([120 150 230]+0)/383;c3 = ([120 150 230]+128)/383;patch([0 1 1 0],[0 0 1 1],c1);patch([0 1 1 1-e 1-e 0+e],[0 0 1 1-e 0+e 0+e],c2);patch([0 0 1 1-e 0+e 0+e],[0 1 1 1-e 1-e 0+e],c3);plot([0 1 1 0 0],[0 0 1 1 0]);disp('+');
  tansig : neural/Transfer Functions/tansig
  "a{1}" : Outport  InitialOutput=[0;0;0;0;0;0;0]
      mask Display: e = 0.06;c1 = [120 230 180]/255;c2 = ([120 230 180]+0)/(256+128);c3 = ([120 230 180]+128)/(256+128);patch([0 1 1 0],[0 0 1 1],c1);patch([0 1 1 1-e 1-e 0+e],[0 0 1 1-e 0+e 0+e],c2);patch([0 0 1 1-e 0+e 0+e],[0 1 1 1-e 1-e 0+e],c3);plot([0 1 1 0 0],[0 0 1 1 0]);
  wires:
  "p{1}"/1 -> Delays 1/1("p{1}")
  Delays 1/1("pd{1,1}") -> "IW{1,1}"/1("pd{1,1}")
  "IW{1,1}"/1("iz{1,1}") -> netsum/1
  "b{1}"/1 -> netsum/2
  netsum/1 -> tansig/1
  tansig/1 -> "a{1}"/1

== system boostObserver_old/Subsystem3/Fault Identification Neural Netowrk/Pattern Recognition Neural Network Reconfig Big Data/Layer 2 ==
  "a{1} " : Inport  PortDimensions=7
      mask Display: e = 0.06;c1 = [120 230 180]/255;c2 = ([120 230 180]+0)/(256+128);c3 = ([120 230 180]+128)/(256+128);patch([0 1 1 0],[0 0 1 1],c1);patch([0 1 1 1-e 1-e 0+e],[0 0 1 1-e 0+e 0+e],c2);patch([0 0 1 1-e 0+e 0+e],[0 1 1 1-e 1-e 0+e],c3);plot([0 1 1 0 0],[0 0 1 1 0]);
  Delays 1 : Subsystem
      mask Display: e = 0.06;c1 = [120 150 230]/255;c2 = ([120 150 230]+0)/383;c3 = ([120 150 230]+128)/383;patch([0 1 1 0],[0 0 1 1],c1);patch([0 1 1 1-e 1-e 0+e],[0 0 1 1-e 0+e 0+e],c2);patch([0 0 1 1-e 0+e 0+e],[0 1 1 1-e 1-e 0+e],c3);plot([0 1 1 0 0],[0 0 1 1 0]);disp('0');
  "LW{2,1}" : Subsystem
      mask Display: e = 0.06;c1 = [120 150 230]/255;c2 = ([120 150 230]+0)/383;c3 = ([120 150 230]+128)/383;patch([0 1 1 0],[0 0 1 1],c1);patch([0 1 1 1-e 1-e 0+e],[0 0 1 1-e 0+e 0+e],c2);patch([0 0 1 1-e 0+e 0+e],[0 1 1 1-e 1-e 0+e],c3);plot([0 1 1 0 0],[0 0 1 1 0]);disp('W');
  "b{2}" : Constant  Value=[0.225431353686377899947501646238379180431365966796875;-0.68129841810407543167826815988519228994846343994140625;0.475110925535897010707486742830951698124408721923828125;-1.6620670436206805842260791905573569238185882568359375;0.019516533547303781259696364713818184100091457366943359375;1.21136502039623739079843289800919592380523681640625]
      mask Display: e = 0.06;c1 = [120 150 230]/255;c2 = ([120 150 230]+0)/383;c3 = ([120 150 230]+128)/383;patch([0 1 1 0],[0 0 1 1],c1);patch([0 1 1 1-e 1-e 0+e],[0 0 1 1-e 0+e 0+e],c2);patch([0 0 1 1-e 0+e 0+e],[0 1 1 1-e 1-e 0+e],c3);plot([0 1 1 0 0],[0 0 1 1 0]);disp('b');
  netsum : Sum  Inputs=2  InputSameDT=on  SaturateOnIntegerOverflow=on  OutDataTypeStr=Inherit: Same as first input
      mask Display: e = 0.06;c1 = [120 150 230]/255;c2 = ([120 150 230]+0)/383;c3 = ([120 150 230]+128)/383;patch([0 1 1 0],[0 0 1 1],c1);patch([0 1 1 1-e 1-e 0+e],[0 0 1 1-e 0+e 0+e],c2);patch([0 0 1 1-e 0+e 0+e],[0 1 1 1-e 1-e 0+e],c3);plot([0 1 1 0 0],[0 0 1 1 0]);disp('+');
  softmax : neural/Transfer Functions/softmax
      settings: SourceProductBaseCode=NN
  "a{2}" : Outport  InitialOutput=[0;0;0;0;0;0]
      mask Display: e = 0.06;c1 = [120 230 180]/255;c2 = ([120 230 180]+0)/(256+128);c3 = ([120 230 180]+128)/(256+128);patch([0 1 1 0],[0 0 1 1],c1);patch([0 1 1 1-e 1-e 0+e],[0 0 1 1-e 0+e 0+e],c2);patch([0 0 1 1-e 0+e 0+e],[0 1 1 1-e 1-e 0+e],c3);plot([0 1 1 0 0],[0 0 1 1 0]);
  wires:
  "a{1} "/1 -> Delays 1/1("p{2}")
  Delays 1/1("pd{2,1}") -> "LW{2,1}"/1("ad{2,1}")
  "LW{2,1}"/1("lz{2,1}") -> netsum/1
  "b{2}"/1 -> netsum/2
  netsum/1 -> softmax/1
  softmax/1 -> "a{2}"/1

== system boostObserver_old/Subsystem3/Fault Identification Neural Netowrk/Pattern Recognition Neural Network Reconfig Big Data/Process Input 1 ==
  x : Inport  PortDimensions=3
      mask Display: e = 0.06;c1 = [120 230 180]/255;c2 = ([120 230 180]+0)/(256+128);c3 = ([120 230 180]+128)/(256+128);patch([0 1 1 0],[0 0 1 1],c1);patch([0 1 1 1-e 1-e 0+e],[0 0 1 1-e 0+e 0+e],c2);patch([0 0 1 1-e 0+e 0+e],[0 1 1 1-e 1-e 0+e],c3);plot([0 1 1 0 0],[0 0 1 1 0]);
  mapminmax : neural/Processing Functions/mapminmax  xmin=[0;0;0]  xmax=[567.909806969347414451476652175;11317.6990431123176676919683814;749.125877625266184622887521982]  ymin=-1  ymax=1
  p : Outport  PortDimensions=3
      mask Display: e = 0.06;c1 = [120 230 180]/255;c2 = ([120 230 180]+0)/(256+128);c3 = ([120 230 180]+128)/(256+128);patch([0 1 1 0],[0 0 1 1],c1);patch([0 1 1 1-e 1-e 0+e],[0 0 1 1-e 0+e 0+e],c2);patch([0 0 1 1-e 0+e 0+e],[0 1 1 1-e 1-e 0+e],c3);plot([0 1 1 0 0],[0 0 1 1 0]);
  wires:
  x/1 -> mapminmax/1
  mapminmax/1 -> p/1

== system boostObserver_old/Subsystem3/Fault Identification Neural Netowrk/Pattern Recognition Neural Network Reconfig Big Data/Process Output 1 ==
  a : Inport  PortDimensions=6
      mask Display: e = 0.06;c1 = [120 230 180]/255;c2 = ([120 230 180]+0)/(256+128);c3 = ([120 230 180]+128)/(256+128);patch([0 1 1 0],[0 0 1 1],c1);patch([0 1 1 1-e 1-e 0+e],[0 0 1 1-e 0+e 0+e],c2);patch([0 0 1 1-e 0+e 0+e],[0 1 1 1-e 1-e 0+e],c3);plot([0 1 1 0 0],[0 0 1 1 0]);
  y : Outport  PortDimensions=6
      mask Display: e = 0.06;c1 = [120 230 180]/255;c2 = ([120 230 180]+0)/(256+128);c3 = ([120 230 180]+128)/(256+128);patch([0 1 1 0],[0 0 1 1],c1);patch([0 1 1 1-e 1-e 0+e],[0 0 1 1-e 0+e 0+e],c2);patch([0 0 1 1-e 0+e 0+e],[0 1 1 1-e 1-e 0+e],c3);plot([0 1 1 0 0],[0 0 1 1 0]);
  wires:
  a/1 -> y/1
